simulink model "throttle"  (R2014b)
settings: Solver=ode3  StartTime=0.0  StopTime=10.0  FixedStep=1  RelTol=1e-3
values from neighbouring files (symbols this model uses):
  alpha_test = alpha(est_points)    [testfile.m]
  p_bef_test = p_bef_thr(est_points)    [testfile.m]
  p_im_test = p_im(est_points)    [testfile.m]
undefined symbols (not defined in the file or in its folder): a_0, a_1, a_2, gamma_air, Newton, R_air, Raphson, T_hat_bef_thr
settings Model: Creator=danfa688  LastModifiedBy=danfa688

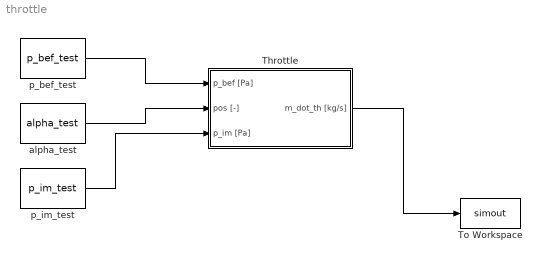
== system throttle ==
  Throttle : Subsystem
  To Workspace : ToWorkspace  VariableName=simout  SaveFormat=Structure With Time  SampleTime=-1
  alpha_test : Constant  Value=alpha_test
  p_bef_test : Constant  Value=p_bef_test
  p_im_test : Constant  Value=p_im_test
  wires:
  p_bef_test/1 -> Throttle/1(p_bef [Pa])
  alpha_test/1 -> Throttle/2(pos [-])
  p_im_test/1 -> Throttle/3(p_im [Pa])
  Throttle/1(m_dot_th [kg/s]) -> To Workspace/1

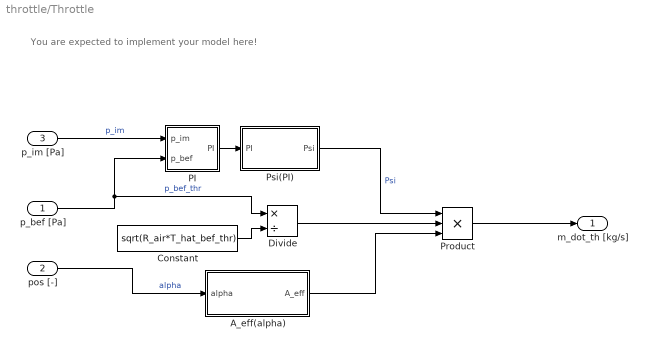
== system throttle/Throttle ==
  note: You are expected to implement your model here!
  p_bef [Pa] : Inport
  pos [-] : Inport  Port=2
  p_im [Pa] : Inport  Port=3
  A_eff(alpha) : Subsystem
  Constant : Constant  Value=sqrt(R_air*T_hat_bef_thr)
  Divide : Product  Inputs=*/
  PI : Subsystem
  Product : Product  Inputs=3
  Psi(PI) : Subsystem
  m_dot_th [kg/s] : Outport
  wires:
  p_im [Pa]/1 -> PI/1(p_im)  "p_im"
  p_bef [Pa]/1 -> PI/2(p_bef), Divide/1  "p_bef_thr"
  pos [-]/1 -> A_eff(alpha)/1(alpha)  "alpha"
  Psi(PI)/1(Psi) -> Product/1  "Psi"
  Product/1 -> m_dot_th [kg/s]/1
  PI/1(PI) -> Psi(PI)/1(PI)
  Constant/1 -> Divide/2
  Divide/1 -> Product/2
  A_eff(alpha)/1(A_eff) -> Product/3

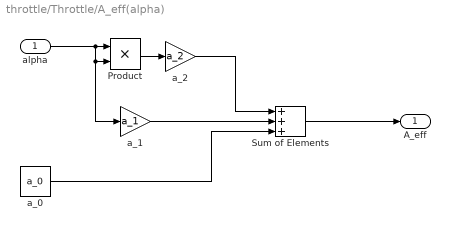
== system throttle/Throttle/A_eff(alpha) ==
  alpha : Inport
  Product : Product
  Sum of Elements : Sum  Inputs=+++
  a_0 : Constant  Value=a_0
  a_1 : Gain  Gain=a_1
  a_2 : Gain  Gain=a_2
  A_eff : Outport
  wires:
  alpha/1 -> a_1/1, Product/2, Product/1
  Sum of Elements/1 -> A_eff/1
  Product/1 -> a_2/1
  a_1/1 -> Sum of Elements/2
  a_2/1 -> Sum of Elements/1
  a_0/1 -> Sum of Elements/3

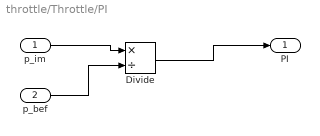
== system throttle/Throttle/PI ==
  p_im : Inport
  p_bef : Inport  Port=2
  Divide : Product  Inputs=*/
  PI : Outport
  wires:
  p_im/1 -> Divide/1
  p_bef/1 -> Divide/2
  Divide/1 -> PI/1

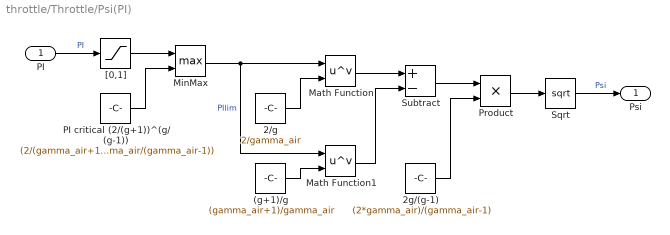
== system throttle/Throttle/Psi(PI) ==
  PI : Inport
  (g+1)/g : Constant  Value=(gamma_air+1)/gamma_air
  2/g : Constant  Value=2/gamma_air
  2g/(g-1) : Constant  Value=(2*gamma_air)/(gamma_air-1)
  Math Function : Math  Operator=pow  SaturateOnIntegerOverflow=on
  Math Function1 : Math  Operator=pow  SaturateOnIntegerOverflow=on
  MinMax : MinMax  Function=max  Inputs=2
  PI critical (2/(g+1))^(g/(g-1)) : Constant  Value=(2/(gamma_air+1))^(gamma_air/(gamma_air-1))
  Product : Product  RndMeth=Zero
  Sqrt : Sqrt  AlgorithmType=Newton-Raphson  SaturateOnIntegerOverflow=on
  Subtract : Sum  Inputs=+-
  "[0,1]" : Saturate  UpperLimit=1  LowerLimit=0
  Psi : Outport
  wires:
  PI/1 -> "[0,1]"/1  "PI"
  PI critical (2/(g+1))^(g/(g-1))/1 -> MinMax/2
  MinMax/1 -> Math Function/1, Math Function1/1  "PIlim"
  2/g/1 -> Math Function/2
  (g+1)/g/1 -> Math Function1/2
  "[0,1]"/1 -> MinMax/1
  Math Function/1 -> Subtract/1
  Math Function1/1 -> Subtract/2
  Subtract/1 -> Product/1
  2g/(g-1)/1 -> Product/2
  Product/1 -> Sqrt/1
  Sqrt/1 -> Psi/1  "Psi"
